simulink model "task2e_model_2015b"  (R2015b)
settings: Solver=VariableStepAuto  StartTime=0.0  StopTime=10.0  RelTol=1e-3
values from neighbouring files (symbols this model uses):
  g = 9.8    [task1.m]    (also in task2c.m; task2e.m = 9.81; task2f.m = 9.81)
  k_1 = linf.k_1    [task2e.m]    (also in task2f.m)
  l = l_hat_linf    [task1.m]    (also in task2c.m = 0.3; task2e.m = 30; task2f.m = 0.3)
  m_s = 0.5    [task2c.m]    (also in task2e.m; task2f.m)
  m_w = linf.m_w    [task2e.m]    (also in task2f.m)
  omega = measurements_3.signals.values(:,5)    [task2e.m]    (also in task2f.m = measurements_4.signals.values(:,5))
  phi = measurements_3.signals.values(:,3)    [task2e.m]    (also in task2f.m = measurements_4.signals.values(:,3))
  V = linf.V    [task2e.m]    (also in task2f.m)
  v_w = measurements_3.signals.values(:,4)    [task2e.m]    (also in task2f.m = measurements_4.signals.values(:,4))
  x_w = measurements_3.signals.values(:,2)    [task2e.m]    (also in task2f.m = measurements_4.signals.values(:,2))
settings Model: Creator=kailintong  LastModifiedBy=kailintong

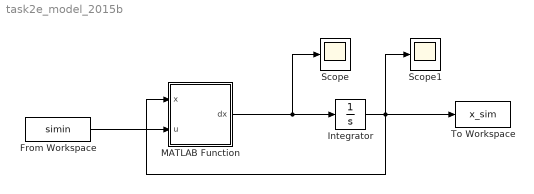
== system task2e_model_2015b ==
  From Workspace : FromWorkspace  VariableName=simin  SampleTime=0
  Integrator : Integrator  InitialCondition=[x_w(1); phi(1); v_w(1); omega(1);]
  MATLAB Function : MATLAB Function  TreatAsAtomicUnit=on
  Scope : Scope
  Scope1 : Scope
  To Workspace : ToWorkspace  VariableName=x_sim  SaveFormat=Structure With Time  SampleTime=-1
  wires:
  MATLAB Function/1(dx) -> Scope/1, Integrator/1
  From Workspace/1 -> MATLAB Function/2(u)
  Integrator/1 -> To Workspace/1, Scope1/1, MATLAB Function/1(x)

== matlab function task2e_model_2015b/MATLAB Function ==
  data: x input; g parameter; dx output; l parameter; u input; m_s parameter; m_w parameter; V parameter; k_1 parameter
function dx = fcn(x,g,l,u, m_s, m_w, V, k_1)
dx = [0;0;0;0];

dx(1) = x(3);
dx(2) = x(4);
dx(3) = (1/(m_w+m_s*(1-cos(x(2))^2)))*(V*u - k_1*x(3) + m_s*l*x(4)^2*sin(x(2)) - m_s*g*sin(x(2))*cos(x(2)));
dx(4) = (1/(1-(m_s/(m_w+m_s))*cos(x(2))^2))*(g*sin(x(2)) - (cos(x(2))/(m_w+m_s))*(V*u-k_1*x(3)) - ((m_s/(m_w+m_s))*l*x(4)^2)*sin(x(2))*cos(x(2)));
